simulink model "lista1_8b"  (R2020b)
settings: Solver=VariableStepAuto  StartTime=0.0  StopTime=10  RelTol=1e-3
settings Model: Creator=lucas  LastModifiedBy=lucas

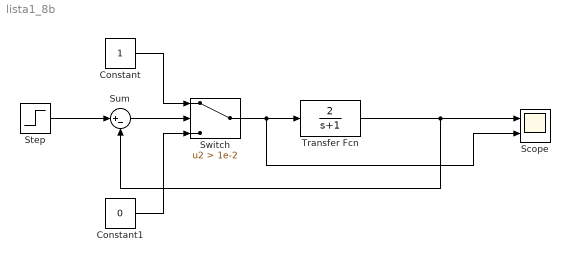
== system lista1_8b ==
  Constant : Constant
  Constant1 : Constant  Value=0
  Scope : Scope  NumInputPorts=2
  Step : Step  Time=0  After=2  SampleTime=0
  Sum : Sum  Inputs=|+-
  Switch : Switch  Criteria=u2 > Threshold  Threshold=1e-2
  Transfer Fcn : TransferFcn  Numerator=[2]  Denominator=[1 1]
  wires:
  Step/1 -> Sum/1
  Sum/1 -> Switch/2
  Constant/1 -> Switch/1
  Constant1/1 -> Switch/3
  Switch/1 -> Transfer Fcn/1, Scope/2
  Transfer Fcn/1 -> Scope/1, Sum/2
